simulink model "main"  (R2021a)
settings: Solver=ode113  StartTime=0.0  StopTime=6*3600  RelTol=1e-13  AbsTol=1e-14
undefined symbols (not defined in the file or in its folder): Const, Earth, initCond, Sensors, Spacecraft
libraries: vrlib x22, aerolibutil x22, SADlibrary x22, dspsrcs4 x14, simulink x7, sharedtransform x5, pid_lib x3, simulink_extras x2, dspmathops x1, sharedutil x1, sharedTrackingLibrary x1
(part 2 of 2)

== system main/Subsystem1/Sun sensor reading4 ==
  True Sun position [body reference frame][km] : Inport  OutDataTypeStr=double  Unit=km
  Atan1 : Trigonometry  Operator=atan2
  Atan2 : Trigonometry  Operator=atan2
  Constant : Constant  Value=0*.5*pi/180*randn(2,1)
  Demux1 : Demux  Outputs=3
  Mux : Mux  Inputs=2
  Normalize Vector : vrlib/Utilities/Normalize Vector  maxzero=0
  Quaternion Rotation : aerolibutil/Quaternion Rotation
  Random Source1 : dspsrcs4/Random Source  SrcType=Gaussian  NormMethod=Ziggurat  CltLength=12  MinVal=0  MaxVal=1  MeanVal=0  VarVal=(.1*pi/180)^2  RepMode=Not repeatable  rawSeed=1  IsInherit=off  SampMode=Discrete  SampTime=Sensors.sunSensorSamplingFreq  SampFrame=2  DataType=Double  OutComplex=Real  OutputFrames=off
  Saturation : Saturate  UpperLimit=60*pi/180  LowerLimit=-60*pi/180
  Sensor orientation : Constant  Value=[cos(pi/4) -sin(pi/4) 0 0]
  Sum : Sum  Inputs=|++
  Sum1 : Sum  Inputs=++|
  Zero-Order Hold : ZeroOrderHold  SampleTime=Sensors.sunSensorSamplingFreq
  Sun angles position [sensor axis] : Outport  OutDataTypeStr=double  Unit=1
  wires:
  True Sun position [body reference frame][km]/1 -> Zero-Order Hold/1
  Sensor orientation/1 -> Quaternion Rotation/1
  Zero-Order Hold/1 -> Normalize Vector/1
  Normalize Vector/1 -> Quaternion Rotation/2
  Quaternion Rotation/1 -> Demux1/1
  Demux1/1 -> Atan2/1
  Demux1/3 -> Atan1/2, Atan2/2
  Demux1/2 -> Atan1/1
  Atan2/1 -> Mux/1
  Atan1/1 -> Mux/2
  Constant/1 -> Sum1/1
  Mux/1 -> Sum1/2
  Saturation/1 -> Sun angles position [sensor axis]/1
  Random Source1/1 -> Sum/2
  Sum/1 -> Saturation/1
  Sum1/1 -> Sum/1

== system main/Subsystem1/Sun sensor reading5 ==
  True Sun position [body reference frame][km] : Inport  OutDataTypeStr=double  Unit=km
  Atan1 : Trigonometry  Operator=atan2
  Atan2 : Trigonometry  Operator=atan2
  Constant : Constant  Value=0*.5*pi/180*randn(2,1)
  Demux1 : Demux  Outputs=3
  Mux : Mux  Inputs=2
  Normalize Vector : vrlib/Utilities/Normalize Vector  maxzero=0
  Quaternion Rotation : aerolibutil/Quaternion Rotation
  Random Source1 : dspsrcs4/Random Source  SrcType=Gaussian  NormMethod=Ziggurat  CltLength=12  MinVal=0  MaxVal=1  MeanVal=0  VarVal=(.1*pi/180)^2  RepMode=Not repeatable  rawSeed=1  IsInherit=off  SampMode=Discrete  SampTime=Sensors.sunSensorSamplingFreq  SampFrame=2  DataType=Double  OutComplex=Real  OutputFrames=off
  Saturation : Saturate  UpperLimit=60*pi/180  LowerLimit=-60*pi/180
  Sensor orientation : Constant  Value=[cos(pi/4) 0 sin(pi/4) 0]
  Sum : Sum  Inputs=|++
  Sum1 : Sum  Inputs=++|
  Zero-Order Hold : ZeroOrderHold  SampleTime=Sensors.sunSensorSamplingFreq
  Sun angles position [sensor axis] : Outport  OutDataTypeStr=double  Unit=1
  wires:
  True Sun position [body reference frame][km]/1 -> Zero-Order Hold/1
  Sensor orientation/1 -> Quaternion Rotation/1
  Zero-Order Hold/1 -> Normalize Vector/1
  Normalize Vector/1 -> Quaternion Rotation/2
  Quaternion Rotation/1 -> Demux1/1
  Demux1/1 -> Atan2/1
  Demux1/3 -> Atan1/2, Atan2/2
  Demux1/2 -> Atan1/1
  Atan2/1 -> Mux/1
  Atan1/1 -> Mux/2
  Constant/1 -> Sum1/1
  Mux/1 -> Sum1/2
  Saturation/1 -> Sun angles position [sensor axis]/1
  Random Source1/1 -> Sum/2
  Sum/1 -> Saturation/1
  Sum1/1 -> Sum/1

== system main/Subsystem1/Sun sensor reading6 ==
  True Sun position [body reference frame][km] : Inport  OutDataTypeStr=double  Unit=km
  Atan1 : Trigonometry  Operator=atan2
  Atan2 : Trigonometry  Operator=atan2
  Constant : Constant  Value=0*.5*pi/180*randn(2,1)
  Demux1 : Demux  Outputs=3
  Mux : Mux  Inputs=2
  Normalize Vector : vrlib/Utilities/Normalize Vector  maxzero=0
  Quaternion Rotation : aerolibutil/Quaternion Rotation
  Random Source1 : dspsrcs4/Random Source  SrcType=Gaussian  NormMethod=Ziggurat  CltLength=12  MinVal=0  MaxVal=1  MeanVal=0  VarVal=(.1*pi/180)^2  RepMode=Not repeatable  rawSeed=1  IsInherit=off  SampMode=Discrete  SampTime=Sensors.sunSensorSamplingFreq  SampFrame=2  DataType=Double  OutComplex=Real  OutputFrames=off
  Saturation : Saturate  UpperLimit=60*pi/180  LowerLimit=-60*pi/180
  Sensor orientation : Constant  Value=[cos(pi/4) 0 -sin(pi/4) 0]
  Sum : Sum  Inputs=|++
  Sum1 : Sum  Inputs=++|
  Zero-Order Hold : ZeroOrderHold  SampleTime=Sensors.sunSensorSamplingFreq
  Sun angles position [sensor axis] : Outport  OutDataTypeStr=double  Unit=1
  wires:
  True Sun position [body reference frame][km]/1 -> Zero-Order Hold/1
  Sensor orientation/1 -> Quaternion Rotation/1
  Zero-Order Hold/1 -> Normalize Vector/1
  Normalize Vector/1 -> Quaternion Rotation/2
  Quaternion Rotation/1 -> Demux1/1
  Demux1/1 -> Atan2/1
  Demux1/3 -> Atan1/2, Atan2/2
  Demux1/2 -> Atan1/1
  Atan2/1 -> Mux/1
  Atan1/1 -> Mux/2
  Constant/1 -> Sum1/1
  Mux/1 -> Sum1/2
  Saturation/1 -> Sun angles position [sensor axis]/1
  Random Source1/1 -> Sum/2
  Sum/1 -> Saturation/1
  Sum1/1 -> Sum/1

== system main/Subsystem3/Sun sensor reading1 ==
  True Sun position [body reference frame][km] : Inport  OutDataTypeStr=double  Unit=km
  Atan1 : Trigonometry  Operator=atan2
  Atan2 : Trigonometry  Operator=atan2
  Constant : Constant  Value=0*.5*pi/180*randn(2,1)
  Demux1 : Demux  Outputs=3
  Mux : Mux  Inputs=2
  Normalize Vector : vrlib/Utilities/Normalize Vector  maxzero=0
  Quaternion Rotation : aerolibutil/Quaternion Rotation
  Random Source1 : dspsrcs4/Random Source  SrcType=Gaussian  NormMethod=Ziggurat  CltLength=12  MinVal=0  MaxVal=1  MeanVal=0  VarVal=(.1*pi/180)^2  RepMode=Not repeatable  rawSeed=1  IsInherit=off  SampMode=Discrete  SampTime=Sensors.sunSensorSamplingFreq  SampFrame=2  DataType=Double  OutComplex=Real  OutputFrames=off
  Saturation : Saturate  UpperLimit=60*pi/180  LowerLimit=-60*pi/180
  Sensor orientation : Constant  Value=[1 0 0 0]
  Sum : Sum  Inputs=|++
  Sum1 : Sum  Inputs=++|
  Zero-Order Hold : ZeroOrderHold  SampleTime=Sensors.sunSensorSamplingFreq
  Sun angles position [sensor axis] : Outport  OutDataTypeStr=double  Unit=1
  wires:
  True Sun position [body reference frame][km]/1 -> Zero-Order Hold/1
  Sensor orientation/1 -> Quaternion Rotation/1
  Zero-Order Hold/1 -> Normalize Vector/1
  Normalize Vector/1 -> Quaternion Rotation/2
  Quaternion Rotation/1 -> Demux1/1
  Demux1/1 -> Atan2/1
  Demux1/3 -> Atan1/2, Atan2/2
  Demux1/2 -> Atan1/1
  Atan2/1 -> Mux/1
  Atan1/1 -> Mux/2
  Constant/1 -> Sum1/1
  Mux/1 -> Sum1/2
  Saturation/1 -> Sun angles position [sensor axis]/1
  Random Source1/1 -> Sum/2
  Sum/1 -> Saturation/1
  Sum1/1 -> Sum/1

== system main/Subsystem3/Sun sensor reading2 ==
  True Sun position [body reference frame][km] : Inport  OutDataTypeStr=double  Unit=km
  Atan1 : Trigonometry  Operator=atan2
  Atan2 : Trigonometry  Operator=atan2
  Constant : Constant  Value=0*.5*pi/180*randn(2,1)
  Demux1 : Demux  Outputs=3
  Mux : Mux  Inputs=2
  Normalize Vector : vrlib/Utilities/Normalize Vector  maxzero=0
  Quaternion Rotation : aerolibutil/Quaternion Rotation
  Random Source1 : dspsrcs4/Random Source  SrcType=Gaussian  NormMethod=Ziggurat  CltLength=12  MinVal=0  MaxVal=1  MeanVal=0  VarVal=(.1*pi/180)^2  RepMode=Not repeatable  rawSeed=1  IsInherit=off  SampMode=Discrete  SampTime=Sensors.sunSensorSamplingFreq  SampFrame=2  DataType=Double  OutComplex=Real  OutputFrames=off
  Saturation : Saturate  UpperLimit=60*pi/180  LowerLimit=-60*pi/180
  Sensor orientation : Constant  Value=[cos(pi/4) sin(pi/4) 0 0]
  Sum : Sum  Inputs=|++
  Sum1 : Sum  Inputs=++|
  Zero-Order Hold : ZeroOrderHold  SampleTime=Sensors.sunSensorSamplingFreq
  Sun angles position [sensor axis] : Outport  OutDataTypeStr=double  Unit=1
  wires:
  True Sun position [body reference frame][km]/1 -> Zero-Order Hold/1
  Sensor orientation/1 -> Quaternion Rotation/1
  Zero-Order Hold/1 -> Normalize Vector/1
  Normalize Vector/1 -> Quaternion Rotation/2
  Quaternion Rotation/1 -> Demux1/1
  Demux1/1 -> Atan2/1
  Demux1/3 -> Atan1/2, Atan2/2
  Demux1/2 -> Atan1/1
  Atan2/1 -> Mux/1
  Atan1/1 -> Mux/2
  Constant/1 -> Sum1/1
  Mux/1 -> Sum1/2
  Saturation/1 -> Sun angles position [sensor axis]/1
  Random Source1/1 -> Sum/2
  Sum/1 -> Saturation/1
  Sum1/1 -> Sum/1

== system main/Subsystem3/Sun sensor reading3 ==
  True Sun position [body reference frame][km] : Inport  OutDataTypeStr=double  Unit=km
  Atan1 : Trigonometry  Operator=atan2
  Atan2 : Trigonometry  Operator=atan2
  Constant : Constant  Value=0*.5*pi/180*randn(2,1)
  Demux1 : Demux  Outputs=3
  Mux : Mux  Inputs=2
  Normalize Vector : vrlib/Utilities/Normalize Vector  maxzero=0
  Quaternion Rotation : aerolibutil/Quaternion Rotation
  Random Source1 : dspsrcs4/Random Source  SrcType=Gaussian  NormMethod=Ziggurat  CltLength=12  MinVal=0  MaxVal=1  MeanVal=0  VarVal=(.1*pi/180)^2  RepMode=Not repeatable  rawSeed=1  IsInherit=off  SampMode=Discrete  SampTime=Sensors.sunSensorSamplingFreq  SampFrame=2  DataType=Double  OutComplex=Real  OutputFrames=off
  Saturation : Saturate  UpperLimit=60*pi/180  LowerLimit=-60*pi/180
  Sensor orientation : Constant  Value=[cos(pi/2) sin(pi/2) 0 0]
  Sum : Sum  Inputs=|++
  Sum1 : Sum  Inputs=++|
  Zero-Order Hold : ZeroOrderHold  SampleTime=Sensors.sunSensorSamplingFreq
  Sun angles position [sensor axis] : Outport  OutDataTypeStr=double  Unit=1
  wires:
  True Sun position [body reference frame][km]/1 -> Zero-Order Hold/1
  Sensor orientation/1 -> Quaternion Rotation/1
  Zero-Order Hold/1 -> Normalize Vector/1
  Normalize Vector/1 -> Quaternion Rotation/2
  Quaternion Rotation/1 -> Demux1/1
  Demux1/1 -> Atan2/1
  Demux1/3 -> Atan1/2, Atan2/2
  Demux1/2 -> Atan1/1
  Atan2/1 -> Mux/1
  Atan1/1 -> Mux/2
  Constant/1 -> Sum1/1
  Mux/1 -> Sum1/2
  Saturation/1 -> Sun angles position [sensor axis]/1
  Random Source1/1 -> Sum/2
  Sum/1 -> Saturation/1
  Sum1/1 -> Sum/1

== system main/Subsystem3/Sun sensor reading4 ==
  True Sun position [body reference frame][km] : Inport  OutDataTypeStr=double  Unit=km
  Atan1 : Trigonometry  Operator=atan2
  Atan2 : Trigonometry  Operator=atan2
  Constant : Constant  Value=0*.5*pi/180*randn(2,1)
  Demux1 : Demux  Outputs=3
  Mux : Mux  Inputs=2
  Normalize Vector : vrlib/Utilities/Normalize Vector  maxzero=0
  Quaternion Rotation : aerolibutil/Quaternion Rotation
  Random Source1 : dspsrcs4/Random Source  SrcType=Gaussian  NormMethod=Ziggurat  CltLength=12  MinVal=0  MaxVal=1  MeanVal=0  VarVal=(.1*pi/180)^2  RepMode=Not repeatable  rawSeed=1  IsInherit=off  SampMode=Discrete  SampTime=Sensors.sunSensorSamplingFreq  SampFrame=2  DataType=Double  OutComplex=Real  OutputFrames=off
  Saturation : Saturate  UpperLimit=60*pi/180  LowerLimit=-60*pi/180
  Sensor orientation : Constant  Value=[cos(pi/4) -sin(pi/4) 0 0]
  Sum : Sum  Inputs=|++
  Sum1 : Sum  Inputs=++|
  Zero-Order Hold : ZeroOrderHold  SampleTime=Sensors.sunSensorSamplingFreq
  Sun angles position [sensor axis] : Outport  OutDataTypeStr=double  Unit=1
  wires:
  True Sun position [body reference frame][km]/1 -> Zero-Order Hold/1
  Sensor orientation/1 -> Quaternion Rotation/1
  Zero-Order Hold/1 -> Normalize Vector/1
  Normalize Vector/1 -> Quaternion Rotation/2
  Quaternion Rotation/1 -> Demux1/1
  Demux1/1 -> Atan2/1
  Demux1/3 -> Atan1/2, Atan2/2
  Demux1/2 -> Atan1/1
  Atan2/1 -> Mux/1
  Atan1/1 -> Mux/2
  Constant/1 -> Sum1/1
  Mux/1 -> Sum1/2
  Saturation/1 -> Sun angles position [sensor axis]/1
  Random Source1/1 -> Sum/2
  Sum/1 -> Saturation/1
  Sum1/1 -> Sum/1

== system main/Subsystem3/Sun sensor reading5 ==
  True Sun position [body reference frame][km] : Inport  OutDataTypeStr=double  Unit=km
  Atan1 : Trigonometry  Operator=atan2
  Atan2 : Trigonometry  Operator=atan2
  Constant : Constant  Value=0*.5*pi/180*randn(2,1)
  Demux1 : Demux  Outputs=3
  Mux : Mux  Inputs=2
  Normalize Vector : vrlib/Utilities/Normalize Vector  maxzero=0
  Quaternion Rotation : aerolibutil/Quaternion Rotation
  Random Source1 : dspsrcs4/Random Source  SrcType=Gaussian  NormMethod=Ziggurat  CltLength=12  MinVal=0  MaxVal=1  MeanVal=0  VarVal=(.1*pi/180)^2  RepMode=Not repeatable  rawSeed=1  IsInherit=off  SampMode=Discrete  SampTime=Sensors.sunSensorSamplingFreq  SampFrame=2  DataType=Double  OutComplex=Real  OutputFrames=off
  Saturation : Saturate  UpperLimit=60*pi/180  LowerLimit=-60*pi/180
  Sensor orientation : Constant  Value=[cos(pi/4) 0 sin(pi/4) 0]
  Sum : Sum  Inputs=|++
  Sum1 : Sum  Inputs=++|
  Zero-Order Hold : ZeroOrderHold  SampleTime=Sensors.sunSensorSamplingFreq
  Sun angles position [sensor axis] : Outport  OutDataTypeStr=double  Unit=1
  wires:
  True Sun position [body reference frame][km]/1 -> Zero-Order Hold/1
  Sensor orientation/1 -> Quaternion Rotation/1
  Zero-Order Hold/1 -> Normalize Vector/1
  Normalize Vector/1 -> Quaternion Rotation/2
  Quaternion Rotation/1 -> Demux1/1
  Demux1/1 -> Atan2/1
  Demux1/3 -> Atan1/2, Atan2/2
  Demux1/2 -> Atan1/1
  Atan2/1 -> Mux/1
  Atan1/1 -> Mux/2
  Constant/1 -> Sum1/1
  Mux/1 -> Sum1/2
  Saturation/1 -> Sun angles position [sensor axis]/1
  Random Source1/1 -> Sum/2
  Sum/1 -> Saturation/1
  Sum1/1 -> Sum/1

== system main/Subsystem3/Sun sensor reading6 ==
  True Sun position [body reference frame][km] : Inport  OutDataTypeStr=double  Unit=km
  Atan1 : Trigonometry  Operator=atan2
  Atan2 : Trigonometry  Operator=atan2
  Constant : Constant  Value=0*.5*pi/180*randn(2,1)
  Demux1 : Demux  Outputs=3
  Mux : Mux  Inputs=2
  Normalize Vector : vrlib/Utilities/Normalize Vector  maxzero=0
  Quaternion Rotation : aerolibutil/Quaternion Rotation
  Random Source1 : dspsrcs4/Random Source  SrcType=Gaussian  NormMethod=Ziggurat  CltLength=12  MinVal=0  MaxVal=1  MeanVal=0  VarVal=(.1*pi/180)^2  RepMode=Not repeatable  rawSeed=1  IsInherit=off  SampMode=Discrete  SampTime=Sensors.sunSensorSamplingFreq  SampFrame=2  DataType=Double  OutComplex=Real  OutputFrames=off
  Saturation : Saturate  UpperLimit=60*pi/180  LowerLimit=-60*pi/180
  Sensor orientation : Constant  Value=[cos(pi/4) 0 -sin(pi/4) 0]
  Sum : Sum  Inputs=|++
  Sum1 : Sum  Inputs=++|
  Zero-Order Hold : ZeroOrderHold  SampleTime=Sensors.sunSensorSamplingFreq
  Sun angles position [sensor axis] : Outport  OutDataTypeStr=double  Unit=1
  wires:
  True Sun position [body reference frame][km]/1 -> Zero-Order Hold/1
  Sensor orientation/1 -> Quaternion Rotation/1
  Zero-Order Hold/1 -> Normalize Vector/1
  Normalize Vector/1 -> Quaternion Rotation/2
  Quaternion Rotation/1 -> Demux1/1
  Demux1/1 -> Atan2/1
  Demux1/3 -> Atan1/2, Atan2/2
  Demux1/2 -> Atan1/1
  Atan2/1 -> Mux/1
  Atan1/1 -> Mux/2
  Constant/1 -> Sum1/1
  Mux/1 -> Sum1/2
  Saturation/1 -> Sun angles position [sensor axis]/1
  Random Source1/1 -> Sum/2
  Sum/1 -> Saturation/1
  Sum1/1 -> Sum/1

== system main/Real physics/Air drag/Air density ==
  note: Because the density is a continuous function it doesn't matter if with an Height equal to a breakpoint value (e.g. =700km) we consider a base height of 700km or a base height of 600km
  Height : Inport
  1-D Lookup Base height : Lookup_n-D  NumberOfTableDimensions=1  BreakpointsForDimension1=Earth.atm_referenceHeight  IndexSearchMethod=Evenly spaced points  BeginIndexSearchUsingPreviousIndexResult=on  Table=Earth.atm_referenceHeight  InterpMethod=Flat  ExtrapMethod=Clip  UseLastTableValue=on  InternalRulePriority=Speed  RndMeth=Simplest  InputSameDT=on
  1-D Lookup Nominal density : Lookup_n-D  NumberOfTableDimensions=1  BreakpointsForDimension1=Earth.atm_referenceHeight  IndexSearchMethod=Evenly spaced points  BeginIndexSearchUsingPreviousIndexResult=on  Table=Earth.atm_nominalDensity  InterpMethod=Flat  InternalRulePriority=Speed  RndMeth=Simplest  InputSameDT=on
  1-D Lookup Scale height : Lookup_n-D  NumberOfTableDimensions=1  BreakpointsForDimension1=Earth.atm_referenceHeight  IndexSearchMethod=Evenly spaced points  BeginIndexSearchUsingPreviousIndexResult=on  Table=Earth.atm_scaleHeight  InterpMethod=Flat  InternalRulePriority=Speed  RndMeth=Simplest  InputSameDT=on
  Divide : Product  Inputs=*/
  Exp : Math  SaturateOnIntegerOverflow=on
  Product : Product
  Sum : Sum  Inputs=-+|
  Air density : Outport
  wires:
  Height/1 -> 1-D Lookup Nominal density/1, 1-D Lookup Scale height/1, 1-D Lookup Base height/1, Sum/1
  1-D Lookup Nominal density/1 -> Product/2
  1-D Lookup Base height/1 -> Sum/2
  Sum/1 -> Divide/1
  1-D Lookup Scale height/1 -> Divide/2
  Divide/1 -> Exp/1
  Product/1 -> Air density/1
  Exp/1 -> Product/1

== system main/Real physics/Magnetic effect (torque only)/Cartesian to polar ==
  Unitary vector [cartesian coord] : Inport
  Atan1 : Trigonometry  Operator=atan2
  Atan2 : Trigonometry  Operator=atan2
  Demux : Demux  Outputs=3
  Sqrt : Sqrt  SaturateOnIntegerOverflow=on
  Square : Math  Operator=square  SaturateOnIntegerOverflow=on
  Square1 : Math  Operator=square  SaturateOnIntegerOverflow=on
  Sum : Sum
  Colatitude - θ : Outport
  Longitude - φ : Outport  Port=2
  wires:
  Demux/2 -> Square1/1, Atan2/1
  Square/1 -> Sum/1
  Square1/1 -> Sum/2
  Atan1/1 -> Colatitude - θ/1
  Sum/1 -> Sqrt/1
  Unitary vector [cartesian coord]/1 -> Demux/1
  Demux/1 -> Square/1, Atan2/2
  Demux/3 -> Atan1/2
  Atan2/1 -> Longitude - φ/1
  Sqrt/1 -> Atan1/1

== system main/Real physics/Rotational dynamic/Euler equations (rigid body)  ==
  note: $\dot\mathbf{\Gamma} = \left[ (-I_z+I_y) \omega_y \omega_z \quad (-I_x+I_z) \omega_z \omega_x \quad \right (-I_y+I_x) \omega_x \omega_y]^T$
      |
      | Please note that
      | $\left[b \quad c \quad a \right] = \text{Cycle_3_vector}\left([a \quad b \quad c]\right)$
  omega [body reference frame] : Inport
  Inertia [body reference frame] : Inport  Port=2  Unit=kg*m^2
  External torque [body reference frame] : Inport  Port=3  Unit=N*m
  Cycle vector{,1..3} (4 alike) : SADlibrary/Cycle vector  SystemSampleTime=-1  VariantActivationTime=update diagram  Latency=0  AutoFrameSizeCalculation=off
  Divide : Product  Inputs=*/
  Product : Product  Inputs=3
  Sum : Sum  Inputs=++|
  Sum1 : Sum  Inputs=|-+
  omega dot [body reference frame] : Outport
  wires:
  Inertia [body reference frame]/1 -> Cycle vector2/1, Divide/2
  External torque [body reference frame]/1 -> Sum/1
  Sum/1 -> Divide/1
  Divide/1 -> omega dot [body reference frame]/1
  omega [body reference frame]/1 -> Cycle vector/1
  Cycle vector2/1 -> Cycle vector3/1, Sum1/1
  Cycle vector3/1 -> Sum1/2
  Cycle vector/1 -> Cycle vector1/1, Product/2
  Cycle vector1/1 -> Product/1
  Sum1/1 -> Product/3
  Product/1 -> Sum/2

== system main/Real physics/Rotational dynamic/Kinematics with quaternions ==
  q : Inport  Unit=1
  omega [body frame] : Inport  Port=2  Unit=rad/s
  Gain1 : Gain  Gain=1/2
  MATLAB Function1 : MATLAB Function  TreatAsAtomicUnit=on
  Matrix Multiply : Product  Multiplication=Matrix(*)
  q dot : Outport
  wires:
  omega [body frame]/1 -> MATLAB Function1/1(omega)
  Gain1/1 -> Matrix Multiply/1
  Matrix Multiply/1 -> q dot/1
  MATLAB Function1/1(Omega) -> Gain1/1
  q/1 -> Matrix Multiply/2

== system main/Real physics/Solar radiation pressure (torque only)/Solar radiation pressure ==
  Distance from the sun : Inport  Unit=km
  1AU [km] : Constant  Value=Const.AU_1
  Divide : Product  Inputs=*/
  Divide1 : Product  Inputs=*/
  Fe [W/m^2] : Constant  Value=Const.Fe
  Product : Product
  Square : Math  Operator=square  SaturateOnIntegerOverflow=on
  c [m/s] : Constant  Value=Const.c
  SRP : Outport  Unit=Pa
  wires:
  1AU [km]/1 -> Divide/1
  Distance from the sun/1 -> Divide/2
  Divide/1 -> Square/1
  Fe [W/m^2]/1 -> Divide1/1
  c [m/s]/1 -> Divide1/2
  Square/1 -> Product/1
  Divide1/1 -> Product/2
  Product/1 -> SRP/1

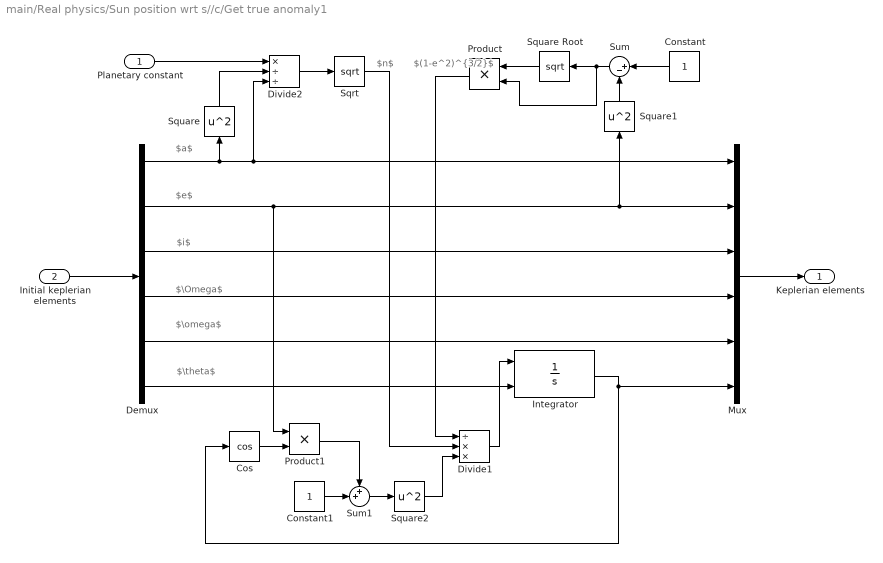
== system main/Real physics/Sun position wrt s//c/Get true anomaly1 ==
  note: $(1-e^2)^{3/2}$
  note: $n$
  note: $\theta$
  note: $\omega$
  note: $\Omega$
  note: $i$
  note: $e$
  note: $a$
  Planetary constant : Inport
  Initial keplerian elements : Inport  Port=2
  Constant : Constant
  Constant1 : Constant
  Cos : Trigonometry  Operator=cos
  Demux : Demux  Outputs=6
  Divide1 : Product  Inputs=/**
  Divide2 : Product  Inputs=*//
  Integrator : Integrator  InitialConditionSource=external
  Mux : Mux  Inputs=6
  Product : Product
  Product1 : Product
  Sqrt : Sqrt  SaturateOnIntegerOverflow=on
  Square : Math  Operator=square  SaturateOnIntegerOverflow=on
  Square Root : Sqrt  SaturateOnIntegerOverflow=on
  Square1 : Math  Operator=square  SaturateOnIntegerOverflow=on
  Square2 : Math  Operator=square  SaturateOnIntegerOverflow=on
  Sum : Sum  Inputs=|+-
  Sum1 : Sum  Inputs=++|
  Keplerian elements : Outport
  wires:
  Initial keplerian elements/1 -> Demux/1
  Mux/1 -> Keplerian elements/1
  Demux/1 -> Square/1, Divide2/3, Mux/1
  Demux/2 -> Mux/2, Square1/1, Product1/1
  Demux/3 -> Mux/3
  Demux/4 -> Mux/4
  Demux/5 -> Mux/5
  Demux/6 -> Integrator/2
  Planetary constant/1 -> Divide2/1
  Square/1 -> Divide2/2
  Divide2/1 -> Sqrt/1
  Sqrt/1 -> Divide1/2
  Constant/1 -> Sum/1
  Square1/1 -> Sum/2
  Sum/1 -> Square Root/1, Product/2
  Square Root/1 -> Product/1
  Product/1 -> Divide1/1
  Cos/1 -> Product1/2
  Square2/1 -> Divide1/3
  Divide1/1 -> Integrator/1
  Constant1/1 -> Sum1/2
  Product1/1 -> Sum1/1
  Sum1/1 -> Square2/1
  Integrator/1 -> Mux/6, Cos/1

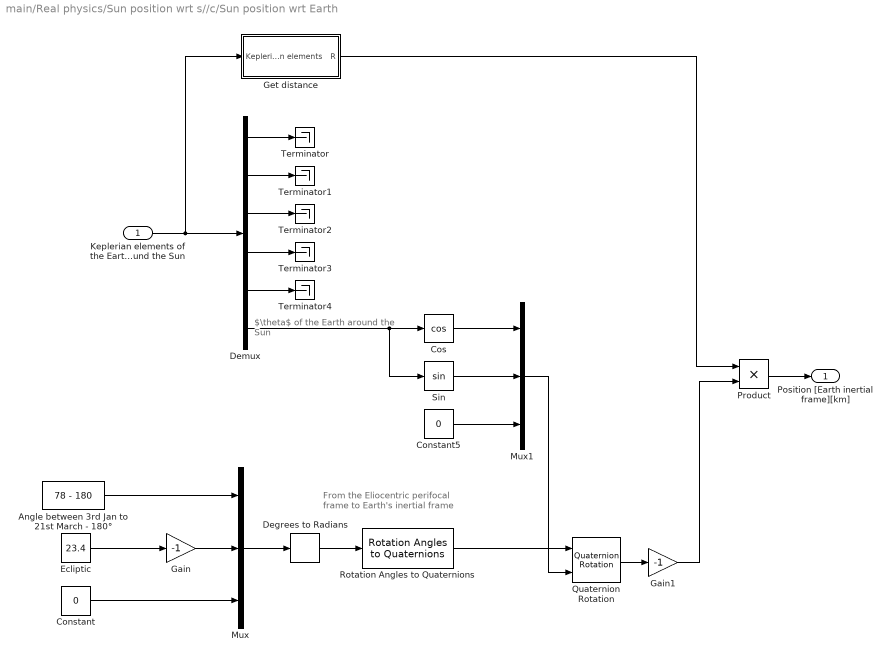
== system main/Real physics/Sun position wrt s//c/Sun position wrt Earth ==
  note: $\theta$ of the Earth around the Sun
  note: From the Eliocentric perifocal frame to Earth's inertial frame
  Keplerian elements of the Earth around the Sun : Inport
  Angle between 3rd Jan to 21st March - 180° : Constant  Value=78 - 180
  Constant : Constant  Value=0
  Constant5 : Constant  Value=0
  Cos : Trigonometry  Operator=cos
  Degrees to Radians : simulink_extras/Transformations/Degrees to Radians
  Demux : Demux  Outputs=6
  Ecliptic : Constant  Value=23.4
  Gain : Gain  Gain=-1
  Gain1 : Gain  Gain=-1
  Get distance : Subsystem
  Mux : Mux  Inputs=3
  Mux1 : Mux  Inputs=3
  Product : Product
  Quaternion Rotation : aerolibutil/Quaternion Rotation
  Rotation Angles to Quaternions : sharedtransform/Rotation Angles to Quaternions  rotationOrder=ZXY  aMode=aMode
      settings: SourceProductBaseCode=AE,PW,DR,MT,UV,VE
  Sin : Trigonometry
  Terminator{,1..4} (5 alike) : Terminator
  Position [Earth inertial frame][km] : Outport  Unit=km
  wires:
  Angle between 3rd Jan to 21st March - 180°/1 -> Mux/1
  Ecliptic/1 -> Gain/1
  Degrees to Radians/1 -> Rotation Angles to Quaternions/1
  Gain/1 -> Mux/2
  Constant/1 -> Mux/3
  Mux/1 -> Degrees to Radians/1
  Mux1/1 -> Quaternion Rotation/2
  Rotation Angles to Quaternions/1 -> Quaternion Rotation/1
  Quaternion Rotation/1 -> Gain1/1
  Gain1/1 -> Product/2
  Keplerian elements of the Earth around the Sun/1 -> Get distance/1(Keplerian elements), Demux/1
  Sin/1 -> Mux1/2
  Constant5/1 -> Mux1/3
  Cos/1 -> Mux1/1
  Demux/6 -> Sin/1, Cos/1
  Get distance/1(R) -> Product/1
  Demux/1 -> Terminator/1
  Demux/2 -> Terminator1/1
  Demux/3 -> Terminator2/1
  Demux/5 -> Terminator4/1
  Demux/4 -> Terminator3/1
  Product/1 -> Position [Earth inertial frame][km]/1

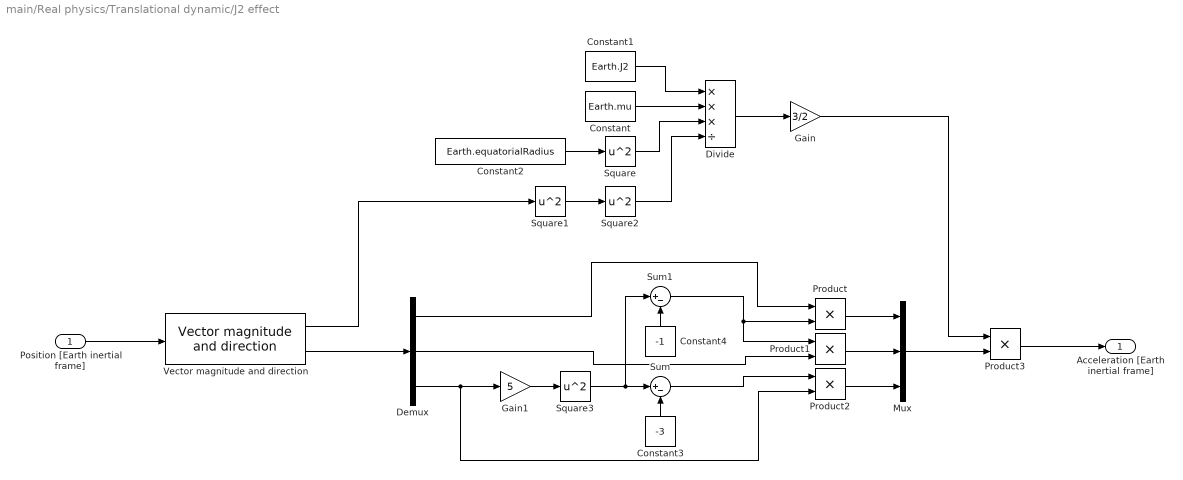
== system main/Real physics/Translational dynamic/J2 effect ==
  Position [Earth inertial frame] : Inport
  Constant : Constant  Value=Earth.mu
  Constant1 : Constant  Value=Earth.J2
  Constant2 : Constant  Value=Earth.equatorialRadius
  Constant3 : Constant  Value=-3
  Constant4 : Constant  Value=-1
  Demux : Demux  Outputs=3
  Divide : Product  Inputs=***/
  Gain : Gain  Gain=3/2
  Gain1 : Gain  Gain=5
  Mux : Mux  Inputs=3
  Product{,1..3} (4 alike) : Product
  Square{,1..3} (4 alike) : Math  Operator=square  SaturateOnIntegerOverflow=on
  Sum : Sum  Inputs=|+-
  Sum1 : Sum  Inputs=|+-
  Vector magnitude and direction : SADlibrary/Vector magnitude and direction  SystemSampleTime=-1  VariantActivationTime=update diagram  Latency=0  AutoFrameSizeCalculation=off
  Acceleration [Earth inertial frame] : Outport
  wires:
  Constant2/1 -> Square/1
  Constant1/1 -> Divide/1
  Constant/1 -> Divide/2
  Square/1 -> Divide/3
  Divide/1 -> Gain/1
  Square1/1 -> Square2/1
  Square2/1 -> Divide/4
  Vector magnitude and direction/1 -> Square1/1
  Position [Earth inertial frame]/1 -> Vector magnitude and direction/1
  Vector magnitude and direction/2 -> Demux/1
  Demux/3 -> Product2/2, Gain1/1
  Gain1/1 -> Square3/1
  Square3/1 -> Sum1/1, Sum/1
  Constant3/1 -> Sum/2
  Constant4/1 -> Sum1/2
  Product/1 -> Mux/1
  Product1/1 -> Mux/2
  Product2/1 -> Mux/3
  Sum1/1 -> Product1/1, Product/2
  Demux/1 -> Product/1
  Demux/2 -> Product1/2
  Sum/1 -> Product2/1
  Mux/1 -> Product3/2
  Product3/1 -> Acceleration [Earth inertial frame]/1
  Gain/1 -> Product3/1

== system main/Real physics/Translational dynamic/Main contribution ==
  Position [Earth inertial frame] : Inport
  Constant : Constant  Value=Earth.mu
  Divide : Product  Inputs=*/
  Gain : Gain  Gain=-1
  Product : Product
  Square : Math  Operator=square  SaturateOnIntegerOverflow=on
  Vector magnitude and direction : SADlibrary/Vector magnitude and direction  SystemSampleTime=-1  VariantActivationTime=update diagram  Latency=0  AutoFrameSizeCalculation=off
  Acceleration [Earth inertial frame] : Outport
  wires:
  Square/1 -> Divide/2
  Product/1 -> Acceleration [Earth inertial frame]/1
  Position [Earth inertial frame]/1 -> Vector magnitude and direction/1
  Divide/1 -> Gain/1
  Constant/1 -> Divide/1
  Vector magnitude and direction/1 -> Square/1
  Vector magnitude and direction/2 -> Product/2
  Gain/1 -> Product/1

== system main/Real physics/Sun position wrt s//c/Sun position wrt Earth/Get distance ==
  note: $\theta$
  note: $e$
  note: $a$
  Keplerian elements : Inport
  Constant : Constant
  Constant3 : Constant
  Cos : Trigonometry  Operator=cos
  Demux : Demux  Outputs=6
  Divide : Product  Inputs=*/
  Product : Product
  Product1 : Product
  Square : Math  Operator=square  SaturateOnIntegerOverflow=on
  Sum : Sum  Inputs=-|+
  Sum1 : Sum  Inputs=+|+
  Terminator : Terminator
  Terminator1 : Terminator
  Terminator2 : Terminator
  R : Outport
  wires:
  Keplerian elements/1 -> Demux/1
  Demux/1 -> Product/1
  Square/1 -> Sum/1
  Sum/1 -> Product/2
  Constant3/1 -> Sum/2
  Product/1 -> Divide/1
  Demux/2 -> Square/1, Product1/1
  Demux/6 -> Cos/1
  Cos/1 -> Product1/2
  Constant/1 -> Sum1/1
  Product1/1 -> Sum1/2
  Sum1/1 -> Divide/2
  Divide/1 -> R/1
  Demux/3 -> Terminator/1
  Demux/5 -> Terminator2/1
  Demux/4 -> Terminator1/1

== matlab function main/Real physics/Solar radiation pressure (torque only)/MATLAB Function ==
  data: sunDir input; F output; SRP input; Spacecraft input; T output
function [F,T] = SRTorque(sunDir,SRP,Spacecraft)
    % Spacecraft data
%     S = {(.1)^2,(.1)^2,(.1)^2,(.1)^2,(.1)^2,(.1)^2, 4.5*(.1)^2,4.5*(.1)^2,4.5*(.1)^2,4.5*(.1)^2};
%     surfNormVec = {[1;0;0],[0;1;0],[0;0;1],[-1;0;0],[0;-1;0],[0;0;-1], [1;0;0],[-1;0;0],[1;0;0],[-1;0;0]};
%     surfPosVec = {.1*[1;0;0],.1*[0;1;0],.1*[0;0;1],.1*[-1;0;0],.1*[0;-1;0],.1*[0;0;-1], .23*[0;1;0],.23*[0;1;0],.23*[0;-1;0],.23*[0;-1;0]};
    rhos = [.5,.5,.5,.5,.5,.5, .8,.8,.8,.8];
    rhod = [.1,.1,.1,.1,.1,.1, .1,.1,.1,.1];
    S = Spacecraft.surfaces_area;
    surfNormVec = Spacecraft.surfaces_normalToSurface;
    surfPosVec = Spacecraft.surfaces_position;
    geometricCenter = Spacecraft.geometricCenter;
    
    F = [0;0;0];
    T = [0;0;0];
    
    for i=1:numel(S)
       sunDir_dot_surfNormVec = dot(sunDir,surfNormVec(:,i));
       S_i = S(i);
       rhos_i = rhos(i);
       rhod_i = rhod(i);
       surfNormVec_i = surfNormVec(:,i);
       surfPosVec_i = surfPosVec(:,i);
       if sunDir_dot_surfNormVec > 0
           F_i = -SRP*S_i*sunDir_dot_surfNormVec*(...
               ( 1-rhos_i )*sunDir + ...
               ( 2/3*rhod_i+2*rhos_i*sunDir_dot_surfNormVec )*surfNormVec_i ...
               );
           F = F + F_i;
           T = T + cross(surfPosVec_i+geometricCenter,F_i);
       end
    end
end

== matlab function main/Real physics/Rotational dynamic/Kinematics with quaternions/MATLAB Function1 ==
  data: omega input size=[3 1]; Omega output size=[4 4]
function Omega = getOmega(omega)
    % Considering the quaternion q = a + i x + j y + k z
    % While in class we used the following convention:
    %   q_vec = [x y z a]'
    % MATLAB use a different convention:
    %   q_vec = [a x y z]'
    % For this reason the following matrix is different from the one we seen
    
    Omega = [         0 -omega(1)  -omega(2) -omega(3) ;
                      0         0   omega(3) -omega(2) ;
                      0         0          0  omega(1) ;
                      0         0          0         0 ];
    Omega = Omega - Omega';
end

== matlab function main/Real physics/Air drag/MATLAB Function ==
  data: F output; rho input; relVel input; T output; Spacecraft input
function [F,T] = getAirTorqueAndForce(rho, relVel, Spacecraft)

F = zeros(3,1);
T = zeros(3,1);

relVelMag = norm(relVel);
relVelDir = relVel/relVelMag;

for i = 1:size(Spacecraft.surfaces_normalToSurface,2)
    N_i = Spacecraft.surfaces_normalToSurface(:,i);
    A_i = Spacecraft.surfaces_area(:,i);
    r_i = Spacecraft.surfaces_position(:,i);
    Cd_i = Spacecraft.surfaces_Cd(i);
    
    F_i = dot(relVelDir,N_i);
    if F_i > 0
       F_i = F_i * 1/2*rho*Cd_i*relVelMag^2*A_i;
    else
       F_i = 0;
    end
    
    F = F - F_i * relVelDir;
    T = T - cross(r_i + Spacecraft.geometricCenter, F_i * relVelDir);
end

== matlab function main/MATLAB Function ==
  data: q input; theta output
function theta = fcn(q)

theta = 2*180/pi*norm(q(2:4));

== matlab function main/Subsystem1/MATLAB Function1 ==
  data: s output size=[2 1]; s1 input; s2 input; s3 input; s4 input; s5 input; s6 input; sensAtt output
function [s,sensAtt] =  getSunSensorReading(s1,s2,s3,s4,s5,s6)
[~,i] = min([sum(s1.^2) sum(s2.^2) sum(s3.^2) sum(s4.^2) sum(s5.^2) sum(s6.^2)]);
switch i
    case 1
        s = s1;
        sensAtt = [1 0 0 0];
    case 2
        s = s2;
        sensAtt = [cos(pi/4) sin(pi/4) 0 0];
    case 3
        s = s3;
        sensAtt = [cos(pi/2) sin(pi/2) 0 0];
    case 4
        s = s4;
        sensAtt = [cos(pi/4) -sin(pi/4) 0 0];
    case 5
        s = s5;
        sensAtt = [cos(pi/4) 0 sin(pi/4) 0];
    case 6
        s = s6;
        sensAtt = [cos(pi/4) 0 -sin(pi/4) 0];
    otherwise
        error("Errore");
end

== matlab function main/MATLAB Function1 ==
  data: SunAngle input; A output; SunSensorAttitudeBF input; SunDirectionECI input; EhiAngle input; EhiSensorAttitudeBF input; EarthDirectionECI input
function A = getAttitude(SunAngle,SunSensorAttitudeBF,SunDirectionECI,EhiAngle,EhiSensorAttitudeBF,EarthDirectionECI)

R = @(q) [     1-2*q(3)^2-2*q(4)^2  2*q(2)*q(3)+2*q(1)*q(4) -2*q(1)*q(3)+2*q(2)*q(4) ;...
           2*q(2)*q(3)-2*q(1)*q(4)      1-2*q(2)^2-2*q(4)^2  2*q(1)*q(2)+2*q(3)*q(4) ;...
           2*q(1)*q(3)+2*q(2)*q(4) -2*q(1)*q(2)+2*q(3)*q(4)      1-2*q(2)^2-2*q(3)^2 ];

%% Sun sensor
% x/z == tan(alphaSun)
% y/z == tan(betaSun)
SunDirectionBF = [tan(SunAngle(1)) tan(SunAngle(2)) 1]';
SunDirectionBF = SunDirectionBF / norm(SunDirectionBF);
SunDirectionBF = R(SunSensorAttitudeBF)*SunDirectionBF;

%% Ehi sensor
EarthDirectionBF = [tan(EhiAngle(1)) tan(EhiAngle(2)) 1]';
EarthDirectionBF = EarthDirectionBF / norm(EarthDirectionBF);
EarthDirectionBF = R(EhiSensorAttitudeBF)*EarthDirectionBF;

sBF = zeros(3);
sBF(:,1) = EarthDirectionBF;
sBF(:,1) = sBF(:,1) / norm(sBF(:,1));
sBF(:,2) = cross(EarthDirectionBF,SunDirectionBF);
sBF(:,2) = sBF(:,2) / norm(sBF(:,2));
sBF(:,3) = cross(sBF(:,1),sBF(:,2));

sECI = zeros(3);
sECI(:,1) = EarthDirectionECI;
sECI(:,1) = sECI(:,1) / norm(sECI(:,1));
sECI(:,2) = cross(EarthDirectionECI,SunDirectionECI);
sECI(:,2) = sECI(:,2) / norm(sECI(:,2));
sECI(:,3) = cross(sECI(:,1),sECI(:,2));

% sBF == R * sECI
A = sBF * sECI';

== matlab function main/Subsystem3/MATLAB Function1 ==
  data: s output size=[2 1]; s1 input; s2 input; s3 input; s4 input; s5 input; s6 input; sensAtt output
function [s,sensAtt] =  getSunSensorReading(s1,s2,s3,s4,s5,s6)
[~,i] = min([sum(s1.^2) sum(s2.^2) sum(s3.^2) sum(s4.^2) sum(s5.^2) sum(s6.^2)]);
switch i
    case 1
        s = s1;
        sensAtt = [1 0 0 0];
    case 2
        s = s2;
        sensAtt = [cos(pi/4) sin(pi/4) 0 0];
    case 3
        s = s3;
        sensAtt = [cos(pi/2) sin(pi/2) 0 0];
    case 4
        s = s4;
        sensAtt = [cos(pi/4) -sin(pi/4) 0 0];
    case 5
        s = s5;
        sensAtt = [cos(pi/4) 0 sin(pi/4) 0];
    case 6
        s = s6;
        sensAtt = [cos(pi/4) 0 -sin(pi/4) 0];
    otherwise
        error("Errore");
end

== matlab function main/MATLAB Function3 ==
  data: earthECI input; angle output; attitude input
function angle = fcn(earthECI,attitude)

R = @(q) [     1-2*q(3)^2-2*q(4)^2  2*q(2)*q(3)+2*q(1)*q(4) -2*q(1)*q(3)+2*q(2)*q(4) ;...
           2*q(2)*q(3)-2*q(1)*q(4)      1-2*q(2)^2-2*q(4)^2  2*q(1)*q(2)+2*q(3)*q(4) ;...
           2*q(1)*q(3)+2*q(2)*q(4) -2*q(1)*q(2)+2*q(3)*q(4)      1-2*q(2)^2-2*q(3)^2 ];

qEarthHorSensor = [cos(pi/2/2) 0 sin(pi/2/2) 0];%[cos(pi/4) -sin(pi/4) 0 0]; %R(qEarthHorSensor)*

earthBF = R(qEarthHorSensor)*R(attitude)*earthECI;

angle = [0;0];
angle(1) = atan2(earthBF(1),earthBF(3));
angle(2) = atan2(earthBF(2),earthBF(3));
